simulink model "ball_sim"  (R2016b)
settings: Solver=ode45  StartTime=0.0  StopTime=1000  RelTol=1e-3  EnableMultiTasking=on
InitFcn:
  | param
undefined symbols (not defined in the file or in its folder): ball_ctrl, drawBallSys, P
settings Model: Creator=beard  LastModifiedBy=Jacob
settings DataIOCC: LimitDataPoints=on  SaveFormat=Array  SignalLoggingSaveFormat=ModelDataLogs
settings OptimizationCC: ExpressionDepthLimit=2147483647  InitFltsAndDblsToZero=on  LifeSpan=inf
settings DebuggingCC: UnderspecifiedInitializationDetection=Classic  MergeDetectMultiDrivingBlocksExec=none  SolverPrmCheckMsg=warning  FcnCallInpInsideContextMsg=warning  StateNameClashWarn=warning  SFUnexpectedBacktrackingDiag=warning  SFNoUnconditionalDefaultTransitionDiag=warning  SFExecutionAtInitializationDiag=none
settings HardwareCC: ProdBitPerPointer=32  ProdBitPerSizeT=32  ProdBitPerPtrDiffT=32  ProdLargestAtomicFloat=None  ProdIntDivRoundTo=Undefined  ProdEndianess=Unspecified  ProdWordSize=32  ProdHWDeviceType=32-bit Generic
settings ModelReferenceCC: PropagateSignalLabelsOutOfModel=off
settings GRTTargetCC: TargetLangStandard=C89/C90 (ANSI)  GeneratePreprocessorConditionals=Disable all  CombineOutputUpdateFcns=off  GRTInterface=on
settings ConfigComp: CovMetricSettings=dw  CovHtmlReporting=on  CovSaveCumulativeToWorkspaceVar=on  CovSaveSingleToWorkspaceVar=on  CovExternalEMLEnable=off

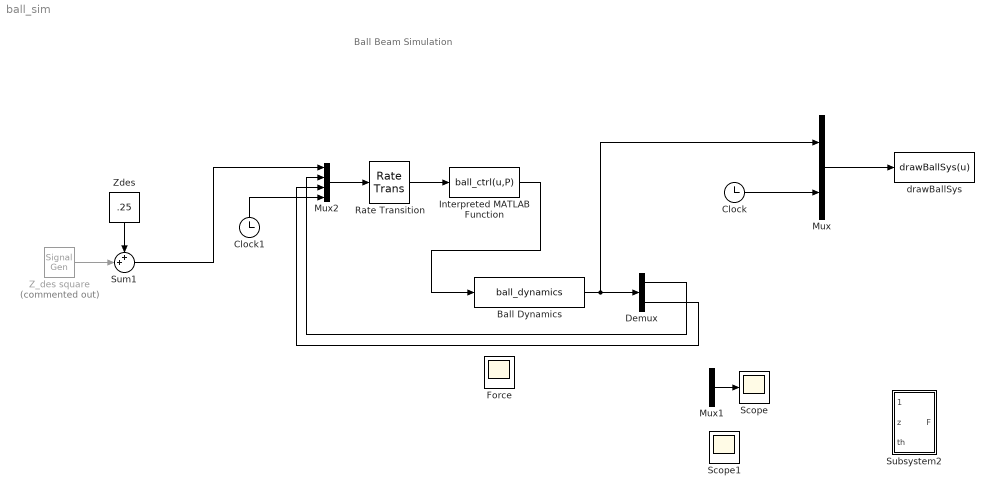
== system ball_sim ==
  note: Ball Beam Simulation
  Ball Dynamics : S-Function  FunctionName=ball_dynamics  Parameters=P  SFunctionDeploymentMode=off  EnableBusSupport=off
  Clock : Clock
  Clock1 : Clock
  Demux : Demux  Outputs=2
  Force : Scope
  Interpreted MATLAB Function : MATLABFcn  MATLABFcn=ball_ctrl(u,P)  OutputDimensions=1
  Mux : Mux  Inputs=2
  Mux1 : Mux  Inputs=2
  Mux2 : Mux
  Rate Transition : RateTransition  OutPortSampleTime=P.Ts
  Scope : Scope
  Scope1 : Scope
  Subsystem2 : Subsystem
  Sum1 : Sum  Inputs=++|
  Z_des square : SignalGenerator  Commented=on  WaveForm=square  Amplitude=.15  Frequency=.01  Units=rad/sec
  Zdes : Constant  Value=.25
  drawBallSys : MATLABFcn  MATLABFcn=drawBallSys(u)  OutputDimensions=0  SampleTime=.5
  wires:
  Mux/1 -> drawBallSys/1
  Clock/1 -> Mux/2
  Ball Dynamics/1 -> Mux/1, Demux/1
  Zdes/1 -> Sum1/1
  Z_des square/1 -> Sum1/2
  Mux1/1 -> Scope/1
  Mux2/1 -> Rate Transition/1
  Sum1/1 -> Mux2/1
  Demux/1 -> Mux2/2
  Demux/2 -> Mux2/3
  Clock1/1 -> Mux2/4
  Rate Transition/1 -> Interpreted MATLAB Function/1
  Interpreted MATLAB Function/1 -> Ball Dynamics/1

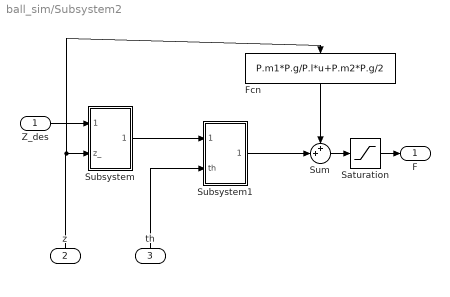
== system ball_sim/Subsystem2 ==
  Z_des : Inport
  z : Inport  Port=2
  th : Inport  Port=3
  Fcn : Fcn  Expr=P.m1*P.g/P.l*u+P.m2*P.g/2
  Saturation : Saturate  UpperLimit=15  LowerLimit=-15
  Subsystem : Subsystem
  Subsystem1 : Subsystem
  Sum : Sum  Inputs=++|
  F : Outport
  wires:
  Fcn/1 -> Sum/1
  Sum/1 -> Saturation/1
  Saturation/1 -> F/1
  Subsystem1/1(Force) -> Sum/2
  Z_des/1 -> Subsystem/1(z_des)
  Subsystem/1(Th_) -> Subsystem1/1(th_des)
  th/1 -> Subsystem1/2(th)
  z/1 -> Fcn/1, Subsystem/2(z_)

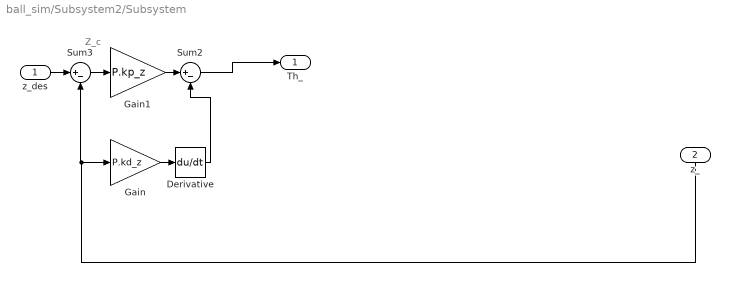
== system ball_sim/Subsystem2/Subsystem ==
  note: Z_c
  z_des : Inport
  z_ : Inport  Port=2
  Derivative : Derivative
  Gain : Gain  Gain=P.kd_z
  Gain1 : Gain  Gain=P.kp_z
  Sum2 : Sum  Inputs=|+-
  Sum3 : Sum  Inputs=|+-
  Th_ : Outport
  wires:
  z_/1 -> Gain/1, Sum3/2
  Sum2/1 -> Th_/1
  Derivative/1 -> Sum2/2
  Gain/1 -> Derivative/1
  Sum3/1 -> Gain1/1
  z_des/1 -> Sum3/1
  Gain1/1 -> Sum2/1

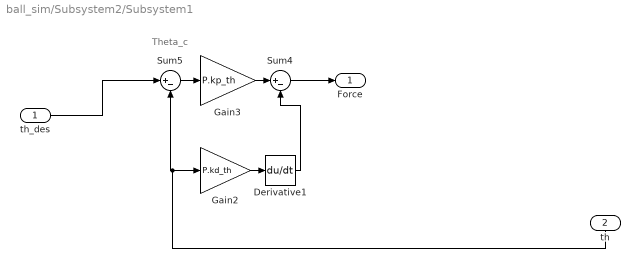
== system ball_sim/Subsystem2/Subsystem1 ==
  note: Theta_c
  th_des : Inport
  th : Inport  Port=2
  Derivative1 : Derivative
  Gain2 : Gain  Gain=P.kd_th
  Gain3 : Gain  Gain=P.kp_th
  Sum4 : Sum  Inputs=|+-
  Sum5 : Sum  Inputs=|+-
  Force : Outport
  wires:
  th/1 -> Gain2/1, Sum5/2
  th_des/1 -> Sum5/1
  Gain3/1 -> Sum4/1
  Sum5/1 -> Gain3/1
  Sum4/1 -> Force/1
  Gain2/1 -> Derivative1/1
  Derivative1/1 -> Sum4/2
